simulink library "hummingbirdLibrary"  (R2017b)
settings: Solver=VariableStepAuto  StartTime=0.0  StopTime=10.0  RelTol=1e-3
libraries: robotcorelib x2
settings Model: Creator=vuwij  LastModifiedBy=vuwij

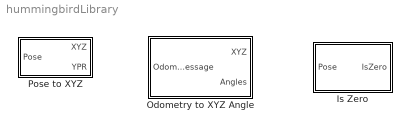
== system hummingbirdLibrary ==
  Is Zero : Subsystem
  Odometry to XYZ Angle : Subsystem
  Pose to XYZ : Subsystem

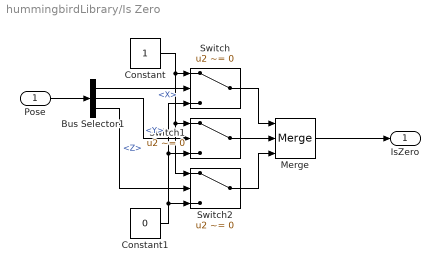
== system hummingbirdLibrary/Is Zero ==
  Pose : Inport
  Bus Selector1 : BusSelector  OutputSignals=Position.X,Position.Y,Position.Z
  Constant : Constant
  Constant1 : Constant  Value=0
  Merge : Merge  Inputs=3
  Switch : Switch  Criteria=u2 ~= 0
  Switch1 : Switch  Criteria=u2 ~= 0
  Switch2 : Switch  Criteria=u2 ~= 0
  IsZero : Outport
  wires:
  Pose/1 -> Bus Selector1/1
  Bus Selector1/2 -> Switch1/2  "<Y>"
  Constant1/1 -> Switch2/3, Switch1/3, Switch/3
  Bus Selector1/1 -> Switch/2  "<X>"
  Bus Selector1/3 -> Switch2/2  "<Z>"
  Switch1/1 -> Merge/2
  Merge/1 -> IsZero/1
  Switch2/1 -> Merge/3
  Switch/1 -> Merge/1
  Constant/1 -> Switch2/1, Switch1/1, Switch/1

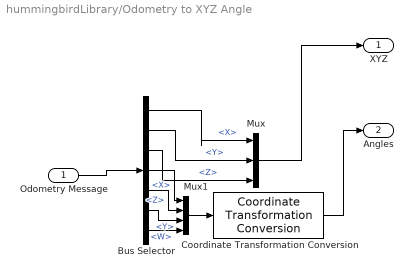
== system hummingbirdLibrary/Odometry to XYZ Angle ==
  Odometry Message : Inport
  Bus Selector : BusSelector  OutputSignals=Pose.Pose.Position.X,Pose.Pose.Position.Y,Pose.Pose.Position.Z,Pose.Pose.Orientation.X,Pose.Pose.Orientation.Z,Pose.Pose.Orientation.Y,Pose.Pose.Orientation.W
  Coordinate Transformation Conversion : robotcorelib/Coordinate Transformation Conversion  InputRepresentation=Quaternion  InputEulerSequence=ZYX  ShowTrVecInputPort=on  OutputRepresentation=Euler Angles  OutputEulerSequence=ZYX  ShowTrVecOutputPort=on  SimulateUsing=Interpreted execution
      settings: SourceProductBaseCode=RO
  Mux : Mux  Inputs=3
  Mux1 : Mux
  XYZ : Outport
  Angles : Outport  Port=2
  wires:
  Odometry Message/1 -> Bus Selector/1
  Mux1/1 -> Coordinate Transformation Conversion/1
  Bus Selector/5 -> Mux1/2  "<Z>"
  Coordinate Transformation Conversion/1 -> Angles/1
  Bus Selector/3 -> Mux/3  "<Z>"
  Bus Selector/7 -> Mux1/4  "<W>"
  Bus Selector/1 -> Mux/1  "<X>"
  Bus Selector/4 -> Mux1/1  "<X>"
  Bus Selector/2 -> Mux/2  "<Y>"
  Bus Selector/6 -> Mux1/3  "<Y>"
  Mux/1 -> XYZ/1

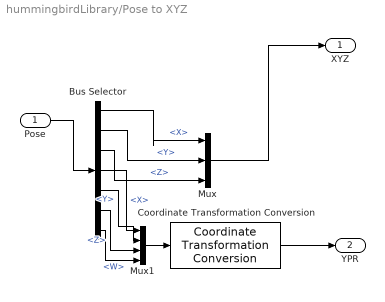
== system hummingbirdLibrary/Pose to XYZ ==
  Pose : Inport
  Bus Selector : BusSelector  OutputSignals=Position.X,Position.Y,Position.Z,Orientation.X,Orientation.Y,Orientation.Z,Orientation.W
  Coordinate Transformation Conversion : robotcorelib/Coordinate Transformation Conversion  InputRepresentation=Quaternion  InputEulerSequence=ZYX  ShowTrVecInputPort=on  OutputRepresentation=Euler Angles  OutputEulerSequence=ZYX  ShowTrVecOutputPort=on  SimulateUsing=Interpreted execution
      settings: SourceProductBaseCode=RO
  Mux : Mux  Inputs=3
  Mux1 : Mux
  XYZ : Outport
  YPR : Outport  Port=2
  wires:
  Mux1/1 -> Coordinate Transformation Conversion/1
  Pose/1 -> Bus Selector/1
  Bus Selector/4 -> Mux1/1  "<X>"
  Bus Selector/6 -> Mux1/3  "<Z>"
  Bus Selector/7 -> Mux1/4  "<W>"
  Bus Selector/3 -> Mux/3  "<Z>"
  Coordinate Transformation Conversion/1 -> YPR/1
  Mux/1 -> XYZ/1
  Bus Selector/2 -> Mux/2  "<Y>"
  Bus Selector/5 -> Mux1/2  "<Y>"
  Bus Selector/1 -> Mux/1  "<X>"
